simulink model "LQR_Lateral_Stability_DLC"  (R2019b)
settings: Solver=FixedStepAuto  StartTime=0.0  StopTime=Time(end)  FixedStep=0.025  RelTol=1e-3
values from neighbouring files (symbols this model uses):
  A = [-(Cf+Cr)/(m*Vx), -1-(lf*Cf-lr*Cr)/(m*Vx^2) ... (first row only)    [LQI_for_LateralStability_LinMod_slipNDyaw.m]    (also in LQR.m; LQR_Model_Initialization.m; LQR_Simulink_testData_DLC.mat = [-4.40211640212  -0.830687830688; 20.8695652174  -5.18678260; LQR_test_data_DLC.mat = [-4.40211640212  -0.830687830688; 20.8695652174  -5.18678260)
  B = [Cf/(m*Vx);(lf*Cf)/Iz]    [LQI_for_LateralStability_LinMod_slipNDyaw.m]    (also in LQR.m; LQR_Model_Initialization.m; LQR_Simulink_testData_DLC.mat = [1.60846560847 15.8608695652]; LQR_test_data_DLC.mat = [1.60846560847 15.8608695652])
  Kc_lqi_t1 = lqi(ss(A,B,C_lqi,D),Q_lqi,R_lqi)    [LQI_for_LateralStability_LinMod_slipNDyaw.m]    (also in LQR_Simulink_testData_DLC.mat = [1.01738471556 0.836422769782 0.0467371713947 -9.99890775876)
settings Model: Creator=Shouvik Chakraborty  LastModifiedBy=shouv
settings DataIOCC: ReturnWorkspaceOutputs=off
settings DebuggingCC: PregeneratedLibrarySubsystemCodeDiagnostic=none  ArithmeticOperatorsInVariantConditions=warning
settings SFSimCC: SimUseLocalCustomCode=off  CustomCodeUndefinedFunction=UseInterfaceOnly
settings RTWCC: RTWUseLocalCustomCode=off

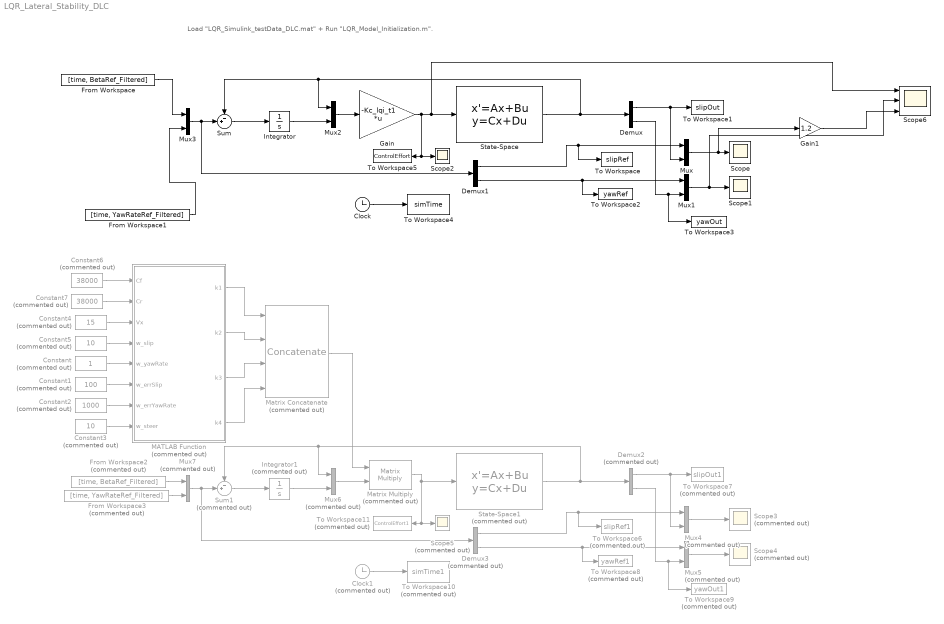
== system LQR_Lateral_Stability_DLC ==
  note: Load "LQR_Simulink_testData_DLC.mat" + Run "LQR_Model_Initialization.m".
  Clock : Clock
  Clock1 : Clock  Commented=on
  Constant : Constant  Commented=on
  Constant1 : Constant  Commented=on  Value=100
  Constant2 : Constant  Commented=on  Value=1000
  Constant3 : Constant  Commented=on  Value=10
  Constant4 : Constant  Commented=on  Value=15
  Constant5 : Constant  Commented=on  Value=10
  Constant6 : Constant  Commented=on  Value=38000
  Constant7 : Constant  Commented=on  Value=38000
  Demux : Demux  Outputs=2
  Demux1 : Demux  Outputs=2
  Demux2 : Demux  Commented=on  Outputs=2
  Demux3 : Demux  Commented=on  Outputs=2
  From Workspace : FromWorkspace  VariableName=[time, BetaRef_Filtered]  SampleTime=0
  From Workspace1 : FromWorkspace  VariableName=[time, YawRateRef_Filtered]  SampleTime=0
  From Workspace2 : FromWorkspace  Commented=on  VariableName=[time, BetaRef_Filtered]  SampleTime=0
  From Workspace3 : FromWorkspace  Commented=on  VariableName=[time, YawRateRef_Filtered]  SampleTime=0
  Gain : Gain  Gain=-Kc_lqi_t1  Multiplication=Matrix(K*u)
  Gain1 : Gain  Gain=1.2
  Integrator : Integrator
  Integrator1 : Integrator  Commented=on
  MATLAB Function : MATLAB Function  Commented=on  TreatAsAtomicUnit=on
  Matrix Concatenate : Concatenate  Commented=on  NumInputs=4  ConcatenateDimension=2
  Matrix Multiply : Product  Commented=on  Multiplication=Matrix(*)
  Mux{,1..3} (4 alike) : Mux  Inputs=2
  Mux{4..7} (4 alike) : Mux  Commented=on  Inputs=2
  Scope : Scope
  Scope1 : Scope
  Scope2 : Scope
  Scope3 : Scope  Commented=on
  Scope4 : Scope  Commented=on
  Scope5 : Scope  Commented=on
  Scope6 : Scope  NumInputPorts=3
  State-Space : StateSpace  A=A  B=B  C=eye(2,2)  D=[0;0]  InitialCondition=0
  State-Space1 : StateSpace  Commented=on  A=A  B=B  C=eye(2,2)  D=[0;0]  InitialCondition=0
  Sum : Sum  Inputs=-+|
  Sum1 : Sum  Commented=on  Inputs=-+|
  To Workspace : ToWorkspace  VariableName=slipRef  SampleTime=-1
  To Workspace1 : ToWorkspace  VariableName=slipOut  SampleTime=-1
  To Workspace10 : ToWorkspace  Commented=on  VariableName=simTime1  SampleTime=-1
  To Workspace11 : ToWorkspace  Commented=on  VariableName=ControlEffort1  SampleTime=-1
  To Workspace2 : ToWorkspace  VariableName=yawRef  SampleTime=-1
  To Workspace3 : ToWorkspace  VariableName=yawOut  SampleTime=-1
  To Workspace4 : ToWorkspace  VariableName=simTime  SampleTime=-1
  To Workspace5 : ToWorkspace  VariableName=ControlEffort  SampleTime=-1
  To Workspace6 : ToWorkspace  Commented=on  VariableName=slipRef1  SampleTime=-1
  To Workspace7 : ToWorkspace  Commented=on  VariableName=slipOut1  SampleTime=-1
  To Workspace8 : ToWorkspace  Commented=on  VariableName=yawRef1  SampleTime=-1
  To Workspace9 : ToWorkspace  Commented=on  VariableName=yawOut1  SampleTime=-1
  wires:
  State-Space/1 -> Sum/1, Mux2/1, Demux/1
  Mux2/1 -> Gain/1
  Integrator/1 -> Mux2/2
  Sum/1 -> Integrator/1
  Mux3/1 -> Demux1/1, Sum/2
  Demux/1 -> Mux/2, To Workspace1/1
  Demux/2 -> To Workspace3/1, Mux1/2
  Demux1/1 -> To Workspace/1, Mux/1
  Demux1/2 -> To Workspace2/1, Mux1/1
  Mux/1 -> Gain1/1, Scope/1
  Mux1/1 -> Scope6/2, Scope1/1
  Gain/1 -> Scope6/1, State-Space/1, Scope2/1, To Workspace5/1
  Clock/1 -> To Workspace4/1
  From Workspace1/1 -> Mux3/2
  Sum1/1 -> Integrator1/1
  Matrix Multiply/1 -> State-Space1/1, Scope5/1, To Workspace11/1
  Demux2/2 -> To Workspace9/1, Mux5/2
  Clock1/1 -> To Workspace10/1
  Mux5/1 -> Scope4/1
  State-Space1/1 -> Sum1/1, Mux6/1, Demux2/1
  Mux4/1 -> Scope3/1
  Demux3/2 -> To Workspace8/1, Mux5/1
  Mux7/1 -> Demux3/1, Sum1/2
  Integrator1/1 -> Mux6/2
  Demux3/1 -> To Workspace6/1, Mux4/1
  Mux6/1 -> Matrix Multiply/2
  From Workspace2/1 -> Mux7/1
  Demux2/1 -> Mux4/2, To Workspace7/1
  From Workspace3/1 -> Mux7/2
  Constant6/1 -> MATLAB Function/1(Cf)
  Constant7/1 -> MATLAB Function/2(Cr)
  Constant4/1 -> MATLAB Function/3(Vx)
  Constant2/1 -> MATLAB Function/7(w_errYawRate)
  Constant3/1 -> MATLAB Function/8(w_steer)
  Constant1/1 -> MATLAB Function/6(w_errSlip)
  Constant5/1 -> MATLAB Function/4(w_slip)
  Constant/1 -> MATLAB Function/5(w_yawRate)
  MATLAB Function/1(k1) -> Matrix Concatenate/1
  MATLAB Function/2(k2) -> Matrix Concatenate/2
  MATLAB Function/3(k3) -> Matrix Concatenate/3
  MATLAB Function/4(k4) -> Matrix Concatenate/4
  Matrix Concatenate/1 -> Matrix Multiply/1
  From Workspace/1 -> Mux3/1
  Gain1/1 -> Scope6/3

== matlab function LQR_Lateral_Stability_DLC/MATLAB Function ==
  data: Cf input; k1 output; Cr input; Vx input; w_slip input; w_yawRate input; w_errSlip input; w_errYawRate input; w_steer input; k2 output; k3 output; k4 output
function [k1,k2,k3,k4] = LQR(Cf, Cr, Vx, w_slip, w_yawRate, w_errSlip, w_errYawRate, w_steer)
coder.extrinsic('ss','lqi')

% Vehicle Configuration parameters
lf=	1.6;
lr=	1.4;
m=1575;
Iz=	2875;

% Code for System Modelling(Continous Time)

A=[-(Cf+Cr)/(m*Vx), -1-(lf*Cf-lr*Cr)/(m*Vx^2);
    -(lf*Cf-lr*Cr)/Iz, -(lf^2*Cf+lr^2*Cr)/(Iz*Vx)];
B=[Cf/(m*Vx);(lf*Cf)/Iz];
C=eye(2);
D=[0];

% Weights for Tuning
Q_lqi=diag([w_slip,w_yawRate,w_errSlip,w_errYawRate]);
R_lqi=[w_steer];

%LQI formulation for Continous Time State space Model.
Klqr=lqi(ss(A,B,C,D),Q_lqi,R_lqi);

k1=-Klqr(1);
k2=-Klqr(2);
k3=-Klqr(3);
k4=-Klqr(4);
